simulink model "bloques"  (R2020a)
settings: Solver=VariableStepAuto  StartTime=0.0  StopTime=800.0  RelTol=1e-3
settings Model: Creator=Royer  LastModifiedBy=Royer

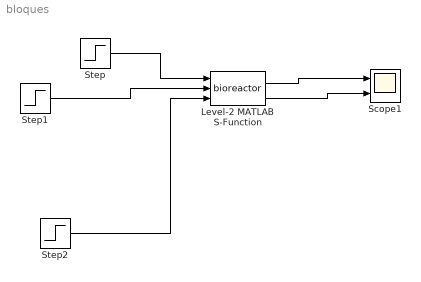
== system bloques ==
  Level-2 MATLAB S-Function : M-S-Function  FunctionName=bioreactor  Parameters=[0.4225;0.0415;2.0535;0.0234]
  Scope1 : Scope  NumInputPorts=2
  Step : Step  Time=0  After=3.3  SampleTime=0
  Step1 : Step  Time=0  Before=0.205  After=0.205  SampleTime=0
  Step2 : Step  Time=0  Before=0.55  After=0.55  SampleTime=0
  wires:
  Step/1 -> Level-2 MATLAB S-Function/1
  Level-2 MATLAB S-Function/1 -> Scope1/1
  Level-2 MATLAB S-Function/2 -> Scope1/2
  Step1/1 -> Level-2 MATLAB S-Function/2
  Step2/1 -> Level-2 MATLAB S-Function/3
